simulink model "sinpwmbanky"  (R2022b)
settings: Solver=VariableStepAuto  StartTime=0.0  StopTime=0.03  RelTol=1e-3
libraries: spsIGBTLib x6, simulink x6, spsDCVoltageSourceLib x1, spsGroundLib x1, spsThreePhaseParallelRLCBranchLib x1, spsThreePhaseVIMeasurementLib x1, spsTriangleGeneratorLib x1, spspowerguiLib x1
settings Model: Creator=doand  LastModifiedBy=doand

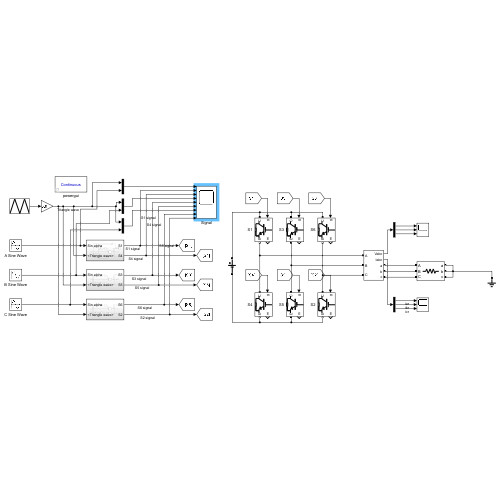
[thumbnail: Simulink's stored preview of the top-level diagram]
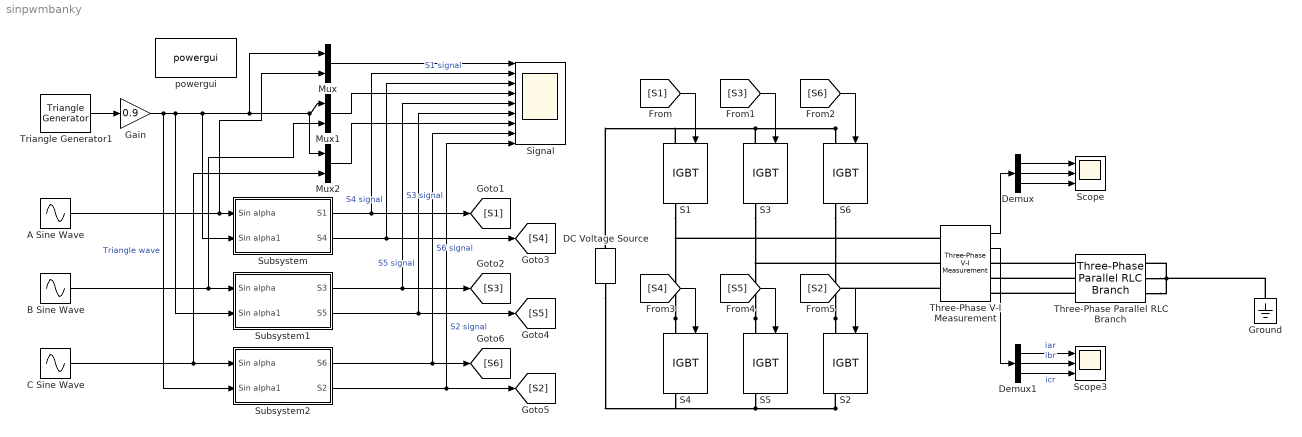
== system sinpwmbanky ==
  A Sine Wave : Sin  Frequency=2*pi*50  SampleTime=0
  B Sine Wave : Sin  Frequency=2*pi*50  Phase=2*pi/3  SampleTime=0
  C Sine Wave : Sin  Frequency=2*pi*50  Phase=-2*pi/3  SampleTime=0
  DC Voltage Source : spsDCVoltageSourceLib/DC Voltage Source  Amplitude=270  Measurements=None
  Demux : Demux  Outputs=3
  Demux1 : Demux  Outputs=3
  Gain : Gain  Gain=0.9
  Ground : spsGroundLib/Ground  LConnTagsString=a
  Mux : Mux  Inputs=2
  Mux1 : Mux  Inputs=2
  Mux2 : Mux  Inputs=2
  S{1..6} (6 alike) : spsIGBTLib/IGBT  Ron=0.001  Lon=0  Vf=1  Tf=1e-6  Tt=2e-6  IC=0  Rs=1e5  Cs=inf  Measurements=on
  Scope : Scope  NumInputPorts=3
  Scope3 : Scope  NumInputPorts=3
  Signal : Scope  NumInputPorts=9
  Subsystem : Subsystem
  Subsystem1 : Subsystem
  Subsystem2 : Subsystem
  Three-Phase Parallel RLC Branch : spsThreePhaseParallelRLCBranchLib/Three-Phase Parallel RLC Branch  LConnTagsString=A|B|C  RConnTagsString=A|B|C  BranchType=R  Resistance=43  Inductance=1e-3  Capacitance=1e-6  Measurements=Branch voltages and currents
  Three-Phase V-I Measurement : spsThreePhaseVIMeasurementLib/Three-Phase V-I Measurement  VoltageMeasurement=phase-to-phase  SetLabelV=off  LabelV=Vabc  Vpu=off  VpuLL=off  CurrentMeasurement=yes  SetLabelI=off  LabelI=Iabc  Ipu=off  Pbase=100e6  Vbase=500e3  OutputType=Complex  PhasorSimulation=off  PSBequivalent=0
  Triangle Generator1 : spsTriangleGeneratorLib/Triangle Generator  Freq=2000*4  Phase=0  Ts=0
  powergui : spspowerguiLib/powergui  Priority=1  SimulationMode=Continuous  SampleTime=50e-6  frequency=60  Iterations=50  frequencyindice=0  Pbase=100e6  ErrMax=1e-4  UnitsV=kV  UnitsW=MW  buscounter=0  FunctionMessages=off  echomessages=off  EnableUseOfTLC=off  CurrentSourceSwitches=off  DisableSnubberDevices=off  DisableRonSwitches=off  DisableVfSwitches=off  DisplayEquations=off  AutomaticDiscreteSolvers=off  SolverType=Tustin/Backward Euler (TBE)  Interpol=off  ExternalGateDelay=off  methode=off  Ts=100  x0status=blocks  SPID=on  SwTol=0  HookPort=off  NonlinearTolerance=1e-4  nMaxIteration=100  ContinueOnMaxIteration=off  RestoreLinks=warning  ResistiveCurrentMeasurement=off  Frange=[0:2:500]  Ylog=off  Xlog=on  ShowGrid=off  save=off  variable=ZData  structure=0  ZoomFFT=off  StartTime=0.0  cycles=1  DisplayStyle=1  fundamental=60  FreqAxis=off  MaxFrequency=1000  frequencyindicesteady=1  RmsSteady=1  display=off
  wires:
  [S1] -> S1/1
  Demux1/1 -> Scope3/1  "iar"
  Demux1/2 -> Scope3/2  "ibr"
  [S2] -> S2/1
  Three-Phase V-I Measurement/1 -> Demux/1
  Demux/2 -> Scope/2
  Demux1/3 -> Scope3/3  "icr"
  Three-Phase V-I Measurement/2 -> Demux1/1
  [S4] -> S4/1
  [S3] -> S3/1
  C Sine Wave/1 -> Subsystem2/1(Sin alpha), Mux2/2
  [S5] -> S5/1
  Demux/3 -> Scope/3
  [S6] -> S6/1
  B Sine Wave/1 -> Mux1/2, Subsystem1/1(Sin alpha)
  A Sine Wave/1 -> Mux/2, Subsystem/1(Sin alpha)
  Demux/1 -> Scope/1
  Subsystem/2(S4) -> [S4], Signal/3  "S4 signal"
  Subsystem1/2(S5) -> Signal/6, [S5]  "S5 signal"
  Subsystem2/2(S2) -> Signal/9, [S2]  "S2 signal"
  Subsystem/1(S1) -> Signal/2, [S1]  "S1 signal"
  Subsystem1/1(S3) -> Signal/5, [S3]  "S3 signal"
  Subsystem2/1(S6) -> Signal/8, [S6]  "S6 signal"
  Triangle Generator1/1 -> Gain/1
  Mux/1 -> Signal/1
  Mux1/1 -> Signal/4
  Mux2/1 -> Signal/7
  Gain/1 -> Subsystem2/2(Sin alpha1), Subsystem1/2(Sin alpha1), Subsystem/2(Sin alpha1), Mux1/1, Mux2/1, Mux/1  "Triangle wave"
  connections:
  S6/LConn1 -- S3/LConn1 -- DC Voltage Source/RConn1 -- S1/LConn1
  S5/LConn1 -- S3/RConn1 -- Three-Phase V-I Measurement/LConn2
  S4/LConn1 -- S1/RConn1 -- Three-Phase V-I Measurement/LConn1
  S2/LConn1 -- S6/RConn1 -- Three-Phase V-I Measurement/LConn3
  S2/RConn1 -- S5/RConn1 -- DC Voltage Source/LConn1 -- S4/RConn1
  Three-Phase Parallel RLC Branch/LConn2 -- Three-Phase V-I Measurement/RConn2
  Three-Phase Parallel RLC Branch/LConn1 -- Three-Phase V-I Measurement/RConn1
  Three-Phase Parallel RLC Branch/LConn3 -- Three-Phase V-I Measurement/RConn3
  Three-Phase Parallel RLC Branch/RConn2 -- Three-Phase Parallel RLC Branch/RConn1 -- Three-Phase Parallel RLC Branch/RConn3 -- Ground/LConn1

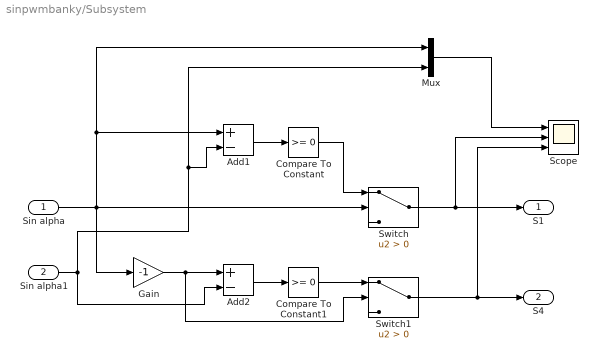
== system sinpwmbanky/Subsystem ==
  Sin alpha : Inport
  Sin alpha1 : Inport  Port=2
  Add1 : Sum  Inputs=+-
  Add2 : Sum  Inputs=+-
  Compare To Constant : simulink/Logic and Bit Operations/Compare To Constant  relop=>=  const=0  OutDataTypeStr=boolean
  Compare To Constant1 : simulink/Logic and Bit Operations/Compare To Constant  relop=>=  const=0  OutDataTypeStr=boolean
  Gain : Gain  Gain=-1
  Mux : Mux  Inputs=2
  Scope : Scope  NumInputPorts=3
  Switch : Switch  Criteria=u2 > Threshold  SaturateOnIntegerOverflow=off  InputSameDT=off
  Switch1 : Switch  Criteria=u2 > Threshold  SaturateOnIntegerOverflow=off  InputSameDT=off
  S1 : Outport
  S4 : Outport  Port=2
  wires:
  Sin alpha/1 -> Gain/1, Switch/2, Mux/1, Add1/1
  Add1/1 -> Compare To Constant/1
  Compare To Constant/1 -> Switch/1
  Switch/1 -> Scope/2, S1/1
  Switch1/1 -> Scope/3, S4/1
  Sin alpha1/1 -> Add2/2, Mux/2, Add1/2
  Add2/1 -> Compare To Constant1/1
  Gain/1 -> Switch1/2, Add2/1
  Compare To Constant1/1 -> Switch1/1
  Mux/1 -> Scope/1

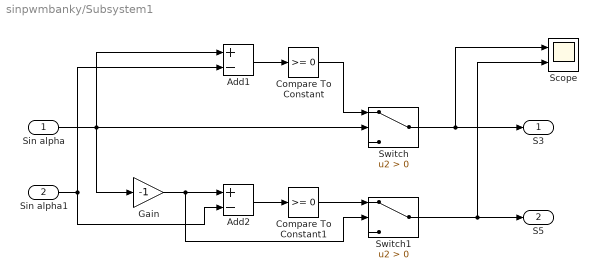
== system sinpwmbanky/Subsystem1 ==
  Sin alpha : Inport
  Sin alpha1 : Inport  Port=2
  Add1 : Sum  Inputs=+-
  Add2 : Sum  Inputs=+-
  Compare To Constant : simulink/Logic and Bit Operations/Compare To Constant  relop=>=  const=0  OutDataTypeStr=boolean
  Compare To Constant1 : simulink/Logic and Bit Operations/Compare To Constant  relop=>=  const=0  OutDataTypeStr=boolean
  Gain : Gain  Gain=-1
  Scope : Scope  NumInputPorts=2
  Switch : Switch  Criteria=u2 > Threshold  SaturateOnIntegerOverflow=off  InputSameDT=off
  Switch1 : Switch  Criteria=u2 > Threshold  SaturateOnIntegerOverflow=off  InputSameDT=off
  S3 : Outport
  S5 : Outport  Port=2
  wires:
  Sin alpha/1 -> Gain/1, Switch/2, Add1/1
  Add1/1 -> Compare To Constant/1
  Compare To Constant/1 -> Switch/1
  Sin alpha1/1 -> Add2/2, Add1/2
  Switch/1 -> Scope/1, S3/1
  Switch1/1 -> Scope/2, S5/1
  Add2/1 -> Compare To Constant1/1
  Gain/1 -> Switch1/2, Add2/1
  Compare To Constant1/1 -> Switch1/1

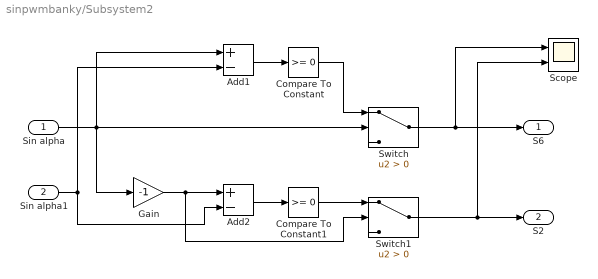
== system sinpwmbanky/Subsystem2 ==
  Sin alpha : Inport
  Sin alpha1 : Inport  Port=2
  Add1 : Sum  Inputs=+-
  Add2 : Sum  Inputs=+-
  Compare To Constant : simulink/Logic and Bit Operations/Compare To Constant  relop=>=  const=0  OutDataTypeStr=boolean
  Compare To Constant1 : simulink/Logic and Bit Operations/Compare To Constant  relop=>=  const=0  OutDataTypeStr=boolean
  Gain : Gain  Gain=-1
  Scope : Scope  NumInputPorts=2
  Switch : Switch  Criteria=u2 > Threshold  SaturateOnIntegerOverflow=off  InputSameDT=off
  Switch1 : Switch  Criteria=u2 > Threshold  SaturateOnIntegerOverflow=off  InputSameDT=off
  S6 : Outport
  S2 : Outport  Port=2
  wires:
  Sin alpha/1 -> Gain/1, Switch/2, Add1/1
  Add1/1 -> Compare To Constant/1
  Compare To Constant/1 -> Switch/1
  Switch/1 -> Scope/1, S6/1
  Switch1/1 -> Scope/2, S2/1
  Sin alpha1/1 -> Add2/2, Add1/2
  Add2/1 -> Compare To Constant1/1
  Gain/1 -> Switch1/2, Add2/1
  Compare To Constant1/1 -> Switch1/1
